simulink model "mod_double_pend"  (R2021a)
settings: Solver=FixedStepAuto  StartTime=0.0  StopTime=10  FixedStep=.01  RelTol=1e-3
model workspace (MAT data in the model file):
  exo_pos_cost_10 : param.Continuous (value not decoded)
values from neighbouring files (symbols this model uses):
  alpha = params.test_25(7,1).Value    [no_exo.m]    (also in non_same_length.m = [15,15]; play_file.m = params.test_22(7,1).Value; play_file22.m = params.test_22(7,1).Value; play_file23.m = params.test_23(7,1).Value)
  beta = params.test_25(5,1).Value    [no_exo.m]    (also in non_same_length.m = [ 1/8 ; 1/8]; play_file.m = params.test_22(5,1).Value; play_file22.m = params.test_22(5,1).Value; play_file23.m = params.test_23(5,1).Value)
  Bn0 = params.test_25(1,1).Value    [no_exo.m]    (also in non_same_length.m = [500  500]; play_file.m = params.test_22(1,1).Value; play_file22.m = params.test_22(1,1).Value; play_file23.m = params.test_23(1,1).Value)
  Bp0 = params.test_25(2,1).Value    [no_exo.m]    (also in non_same_length.m = [500  500]; play_file.m = params.test_22(2,1).Value; play_file22.m = params.test_22(2,1).Value; play_file23.m = params.test_23(2,1).Value)
  dampener = [100, 0; 0, 100]    [no_exo.m]    (also in non_same_length.m; play_file.m; play_file22.m; play_file23.m)
  Dm1 = [1000,0;0,103.228187679703]    [no_exo.m]    (also in non_same_length.m = [30,0;0,30]; play_file.m = [30,0;0,30]; play_file22.m = [300,0;0,300]; play_file23.m = [30,0;0,30])
  exo_sat = 0.0    (= 0)    [no_exo.m]    (also in non_same_length.m = 150; play_file.m = 150; play_file22.m = 150; play_file23.m = 150)
  gamma = params.test_25(9,1).Value    [no_exo.m]    (also in non_same_length.m = [15,15]; play_file.m = params.test_22(9,1).Value; play_file22.m = params.test_22(9,1).Value; play_file23.m = params.test_23(9,1).Value)
  human_sat = 150    [no_exo.m]    (also in non_same_length.m = 30; play_file.m = 30; play_file22.m = 30; play_file23.m = 200)
  Ked = [ 50, 0; 0, 50]    [no_exo.m]    (also in non_same_length.m; play_file.m; play_file22.m; play_file23.m)
  Kem = [ 50, 0; 0, 50]    [no_exo.m]    (also in non_same_length.m; play_file.m; play_file22.m; play_file23.m)
  Km1 = [1000,0;0,1000]    [no_exo.m]    (also in non_same_length.m = [30, 0; 0 30]; play_file.m = [30, 0; 0 30]; play_file22.m = [300, 0; 0 300]; play_file23.m = [30, 0; 0 30])
  Kn0 = params.test_25(3,1).Value    [no_exo.m]    (also in non_same_length.m = [500  500]; play_file.m = params.test_22(3,1).Value; play_file22.m = params.test_22(3,1).Value; play_file23.m = params.test_23(3,1).Value)
  Kp0 = params.test_25(4,1).Value    [no_exo.m]    (also in non_same_length.m = [500 500]; play_file.m = params.test_22(4,1).Value; play_file22.m = params.test_22(4,1).Value; play_file23.m = params.test_23(4,1).Value)
  l = [0.324, 0.3900]    [myStateTransitionFcn.m]
  lambda2 = params.test_25(6,1).Value    [no_exo.m]    (also in non_same_length.m = [1.2, 0; 0 1.25]; play_file.m = params.test_22(6,1).Value; play_file22.m = params.test_22(6,1).Value; play_file23.m = params.test_23(6,1).Value)
  le = [0.324, 0.3900]    [no_exo.m]    (also in non_same_length.m; play_file.m; play_file22.m; play_file23.m)
  lh = [0.324, 0.3900]    [no_exo.m]    (also in non_same_length.m; play_file.m; play_file22.m; play_file23.m)
  Md = [10.0, 0; 0, 10.0]    [no_exo.m]    (also in non_same_length.m; play_file.m; play_file22.m; play_file23.m)
  me = [ 2.11, 1.28]  + mh    [no_exo.m]    (also in non_same_length.m; play_file.m; play_file22.m; play_file23.m)
  mh = [11.824, 3.848]    [no_exo.m]    (also in non_same_length.m; play_file.m; play_file22.m; play_file23.m)
  rho2 = params.test_25(8,1).Value    [no_exo.m]    (also in non_same_length.m = [100, 0; 0, 450]; play_file.m = params.test_22(8,1).Value; play_file22.m = params.test_22(8,1).Value; play_file23.m = params.test_23(8,1).Value)
  spring = [100, 0; 0, 100]    [no_exo.m]    (also in non_same_length.m; play_file.m; play_file22.m; play_file23.m)
undefined symbols (not defined in the file or in its folder): l1, l2, me2
libraries: simulink x4, sharedTrackingLibrary x1, robotcorelib x1
(part 2 of 2)

== matlab function mod_double_pend/addmittance2/MATLAB Function ==
  data: Tid input; K output; Th input; qd input; B output
function [K,B] = fcn(Tid, Th, qd)

Kp0 = [75 0; 0 25];
Kn0 = [50 0; 0 50];
Bp0 = [75 0; 0 25];
Bn0 = [50 0; 0 50];
beta_p = 3;
beta_n = 3;
alpha_p = 0.5;
alpha_n = 0.5;

intention = sign(Th) == sign(qd);
change = abs(Th/Tid);

K = eye(size(intention,1));
B = eye(size(intention,1));
count = 1;
my_intention = [0;0];


for ii =  1:length(intention)
   if intention(ii)
        K(count,count) = Kp0(count,count) + beta_p*change(count);
        B(count,count) = Bp0(count,count) + alpha_p*change(count);
   else
       K(count,count) = Kn0(count,count) - beta_n*change(count);
       B(count,count) = Bn0(count,count) - alpha_n*change(count);
   end
   my_intention(count) = 0;
   count= count + 1;
   

end


end
